simulink model "rectifier_buck_converter"  (R2021a)
settings: Solver=VariableStepAuto  StartTime=0.0  StopTime=10.0  RelTol=1e-3
libraries: spsDiodeLib x7, spsACVoltageSourceLib x3, spsVoltageMeasurementLib x3, spsCurrentMeasurementLib x2, spsDCMachineLib x1, spsDCVoltageSourceLib x1, spsIGBTLib x1, dspstat3 x1, spsSeriesRLCBranchLib x1, spspowerguiLib x1
settings Model: Creator=DELL  LastModifiedBy=DELL

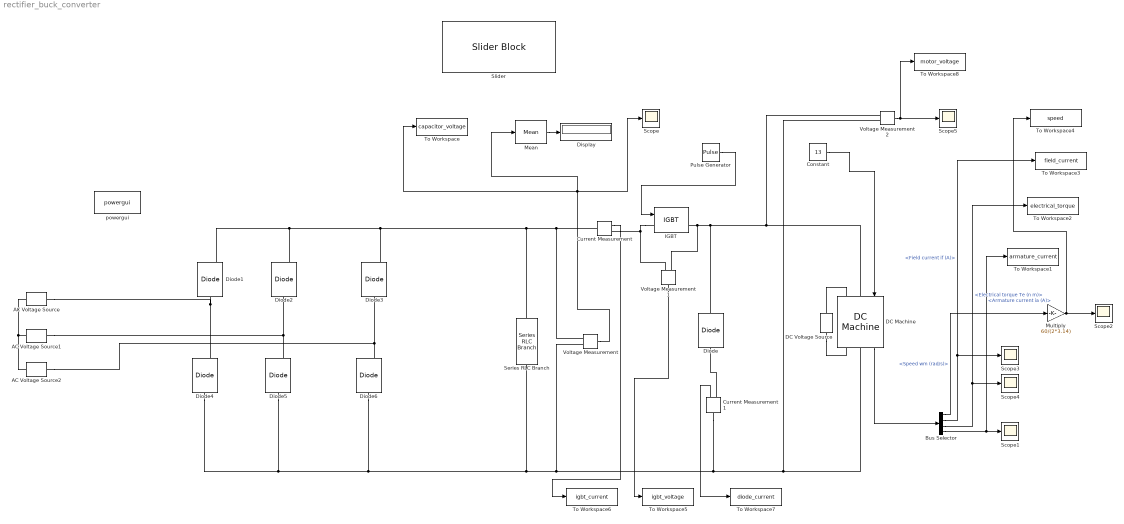
== system rectifier_buck_converter ==
  AC Voltage Source : spsACVoltageSourceLib/AC Voltage Source  Amplitude=135  Phase=0  Frequency=50  SampleTime=0  Measurements=None  BusType=swing  Pref=10e3  Qref=0  Qmin=-inf  Qmax=+inf
  AC Voltage Source1 : spsACVoltageSourceLib/AC Voltage Source  Amplitude=135  Phase=120  Frequency=50  SampleTime=0  Measurements=None  BusType=swing  Pref=10e3  Qref=0  Qmin=-inf  Qmax=+inf
  AC Voltage Source2 : spsACVoltageSourceLib/AC Voltage Source  Amplitude=135  Phase=240  Frequency=50  SampleTime=0  Measurements=None  BusType=swing  Pref=10e3  Qref=0  Qmin=-inf  Qmax=+inf
  Bus Selector : BusSelector  OutputSignals=Speed wm (rad/s),Field current if (A),Electrical torque Te (n m),Armature current ia (A)
  Constant : Constant  Value=13
  Current Measurement : spsCurrentMeasurementLib/Current Measurement  PhasorSimulation=off  OutputType=Complex  PSBequivalent=0
  Current Measurement1 : spsCurrentMeasurementLib/Current Measurement  PhasorSimulation=off  OutputType=Complex  PSBequivalent=0
  DC Machine : spsDCMachineLib/DC Machine  PresetModel=No  MechanicalLoad=Torque TL  FieldType=Wound  ShowDetailedParameters=on  MeasurementBus=off  RLa="[ 0.8  0.012]"  RLf="[ 240  120]"  Laf=1.8  MachineConstant=Back-emf constant (V/rpm)  Ke=200/1500  Kt=1.8  J=1  Bm=0  Tf=0  w0=1  Ifinit=0.583333332757606  TsPowergui=0  TsBlock=-1
  DC Voltage Source : spsDCVoltageSourceLib/DC Voltage Source  Amplitude=140  Measurements=None
  Diode : spsDiodeLib/Diode  Ron=0.001  Lon=0  Vf=0.8  IC=0  UseSnubber=0  Rs=500  Cs=250e-9  Measurements=off
  Diode{1..6} (6 alike) : spsDiodeLib/Diode  Ron=0.001  Lon=0  Vf=0.8  IC=0  UseSnubber=0  Rs=500  Cs=250e-9  Measurements=on
  Display : Display
  IGBT : spsIGBTLib/IGBT  Ron=0.001  Lon=0  Vf=1  Tf=1e-6  Tt=2e-6  IC=0  Rs=1e5  Cs=inf  Measurements=on
  Mean : dspstat3/Mean  run=off  InputProcessing=Columns as channels (frame based)  reset_popup=None  directionMode=Each column  dimension=1  roiEnable=off  roiType=Rectangles  roiPortion=Entire ROI  roiOutput=Individual statistics for each ROI  roiFlag=off  roundingMode=Floor  overflowMode=off  outputDataTypeStr=Inherit: Same as accumulator  outputMin=[]  outputMax=[]  outputLastDataTypeStr=Inherit: Same as accumulator
  Multiply : Gain  Gain=60/(2*3.14)
  Pulse Generator : DiscretePulseGenerator  PulseType=Time based  Amplitude=10  Period=1/10000  PulseWidth=80
  Scope{,1..5} (6 alike) : Scope
  Series RLC Branch : spsSeriesRLCBranchLib/Series RLC Branch  LConnTagsString=__new0  RConnTagsString=__new0  BranchType=C  Resistance=1  Inductance=1e-3  SetiL0=off  InitialCurrent=0  Capacitance=800e-6  Setx0=off  InitialVoltage=0  Measurements=None
  Slider : SliderBlock
  To Workspace : ToWorkspace  VariableName=capacitor_voltage  SaveFormat=Timeseries  SampleTime=-1
  To Workspace1 : ToWorkspace  VariableName=armature_current  SaveFormat=Timeseries  SampleTime=-1
  To Workspace2 : ToWorkspace  VariableName=electrical_torque  SaveFormat=Timeseries  SampleTime=-1
  To Workspace3 : ToWorkspace  VariableName=field_current  SaveFormat=Timeseries  SampleTime=-1
  To Workspace4 : ToWorkspace  VariableName=speed  SaveFormat=Timeseries  SampleTime=-1
  To Workspace5 : ToWorkspace  VariableName=igbt_voltage  SaveFormat=Timeseries  SampleTime=-1
  To Workspace6 : ToWorkspace  VariableName=igbt_current  SaveFormat=Timeseries  SampleTime=-1
  To Workspace7 : ToWorkspace  VariableName=diode_current  SaveFormat=Timeseries  SampleTime=-1
  To Workspace8 : ToWorkspace  VariableName=motor_voltage  SaveFormat=Timeseries  SampleTime=-1
  Voltage Measurement : spsVoltageMeasurementLib/Voltage Measurement  PhasorSimulation=off  OutputType=Complex  PSBequivalent=0
  Voltage Measurement1 : spsVoltageMeasurementLib/Voltage Measurement  PhasorSimulation=off  OutputType=Complex  PSBequivalent=0
  Voltage Measurement2 : spsVoltageMeasurementLib/Voltage Measurement  PhasorSimulation=off  OutputType=Complex  PSBequivalent=0
  powergui : spspowerguiLib/powergui  Priority=1  SimulationMode=Continuous  SampleTime=50e-6  frequency=60  Iterations=50  frequencyindice=50  Pbase=100e6  ErrMax=1e-4  UnitsV=kV  UnitsW=MW  buscounter=0  FunctionMessages=off  echomessages=off  EnableUseOfTLC=off  CurrentSourceSwitches=off  DisableSnubberDevices=off  DisableRonSwitches=off  DisableVfSwitches=off  DisplayEquations=off  AutomaticDiscreteSolvers=off  SolverType=Tustin/Backward Euler (TBE)  Interpol=off  ExternalGateDelay=off  methode=off  Ts=100  x0status=blocks  SPID=on  SwTol=0  HookPort=off  NonlinearTolerance=1e-4  nMaxIteration=100  ContinueOnMaxIteration=off  RestoreLinks=warning  ResistiveCurrentMeasurement=off  Frange=[0:2:500]  Ylog=off  Xlog=on  ShowGrid=off  save=off  variable=ZData  structure=0  ZoomFFT=off  StartTime=0.0  cycles=1  DisplayStyle=1  fundamental=60  FreqAxis=off  MaxFrequency=1000  frequencyindicesteady=1  RmsSteady=1  display=off
  wires:
  Current Measurement1/1 -> To Workspace7/1
  Voltage Measurement1/1 -> To Workspace5/1
  Mean/1 -> Display/1
  DC Machine/1 -> Bus Selector/1
  Bus Selector/1 -> Multiply/1  "<Speed wm (rad/s)>"
  Pulse Generator/1 -> IGBT/1
  Bus Selector/4 -> To Workspace1/1, Scope1/1  "<Armature current ia (A)>"
  Voltage Measurement/1 -> Mean/1, Scope/1, To Workspace/1
  Constant/1 -> DC Machine/1
  Bus Selector/3 -> To Workspace2/1, Scope4/1  "<Electrical torque Te (n m)>"
  Bus Selector/2 -> To Workspace3/1, Scope3/1  "<Field current if (A)>"
  Current Measurement/1 -> To Workspace6/1
  Voltage Measurement2/1 -> To Workspace8/1, Scope5/1
  Multiply/1 -> To Workspace4/1, Scope2/1
  connections:
  Diode4/LConn1 -- Diode5/LConn1 -- Diode6/LConn1 -- Series RLC Branch/RConn1 -- Voltage Measurement/LConn2 -- Current Measurement1/LConn1 -- Voltage Measurement2/LConn2 -- DC Machine/RConn1
  Voltage Measurement/LConn1 -- Current Measurement/LConn1 -- Diode2/RConn1 -- Diode1/RConn1 -- Diode3/RConn1 -- Series RLC Branch/LConn1
  IGBT/LConn1 -- Voltage Measurement1/LConn2 -- Current Measurement/RConn1
  Current Measurement1/RConn1 -- Diode/LConn1
  DC Voltage Source/LConn1 -- DC Machine/RConn2
  DC Voltage Source/RConn1 -- DC Machine/LConn2
  Diode4/RConn1 -- AC Voltage Source/RConn1 -- Diode1/LConn1
  Diode5/RConn1 -- Diode2/LConn1 -- AC Voltage Source1/RConn1
  Diode6/RConn1 -- AC Voltage Source2/RConn1 -- Diode3/LConn1
  AC Voltage Source/LConn1 -- AC Voltage Source2/LConn1 -- AC Voltage Source1/LConn1
  Voltage Measurement1/LConn1 -- DC Machine/LConn1 -- Voltage Measurement2/LConn1 -- Diode/RConn1 -- IGBT/RConn1
